simulink model "Monitor"  (R2020a)
settings: Solver=FixedStepAuto  StartTime=0.0  StopTime=4  FixedStep=0.01  RelTol=1e-3
undefined symbols (not defined in the file): a03c, a5a6, b93b39085928, BLE_Receive, Button, Case_of_study, Ci, Data_Display, Data_Display1, F4, intentBLE, Ri, Size_received, Slider, tau1
libraries: androiduilib x14, simulink x4, androidcommunicationlib x2, dspswit3 x2, hdlsllib x1
settings Model: Creator=luisi  LastModifiedBy=luisi
settings OptimizationCC: EnhancedBackFolding=on  PassReuseOutputArgsAs=Individual arguments  ZeroExternalMemoryAtStartup=off  ZeroInternalMemoryAtStartup=off  MaxStackSize=64  OptimizeBlockOrder=speed  DifferentSizesBufferReuse=on  OptimizationCustomize=off  EfficientTunableParamExpr=on
settings DebuggingCC: ParameterTunabilityLossMsg=error
settings HardwareCC: ProdBitPerPointer=32  ProdBitPerSizeT=32  ProdBitPerPtrDiffT=32  ProdLargestAtomicInteger=Long  ProdLargestAtomicFloat=Double  ProdWordSize=32  ProdHWDeviceType=ARM Compatible->ARM Cortex
settings SFSimCC: MATLABDynamicMemAlloc=off
settings RTWCC: SystemTargetFile=ert.tlc  HardwareBoard=Android Device  TemplateMakefile=ert_default_tmf  RTWVerbose=off  Toolchain=Android SDK/NDK Tools
settings CodeAppCC: ForceParamTrailComments=on  IgnoreCustomStorageClasses=off  OperatorAnnotations=on  SimulinkDataObjDesc=on  SFDataObjDesc=on  InsertBlockDesc=on
settings ERTTargetCC: SupportContinuousTime=on  ExtModeMexArgs='192.168.0.106'

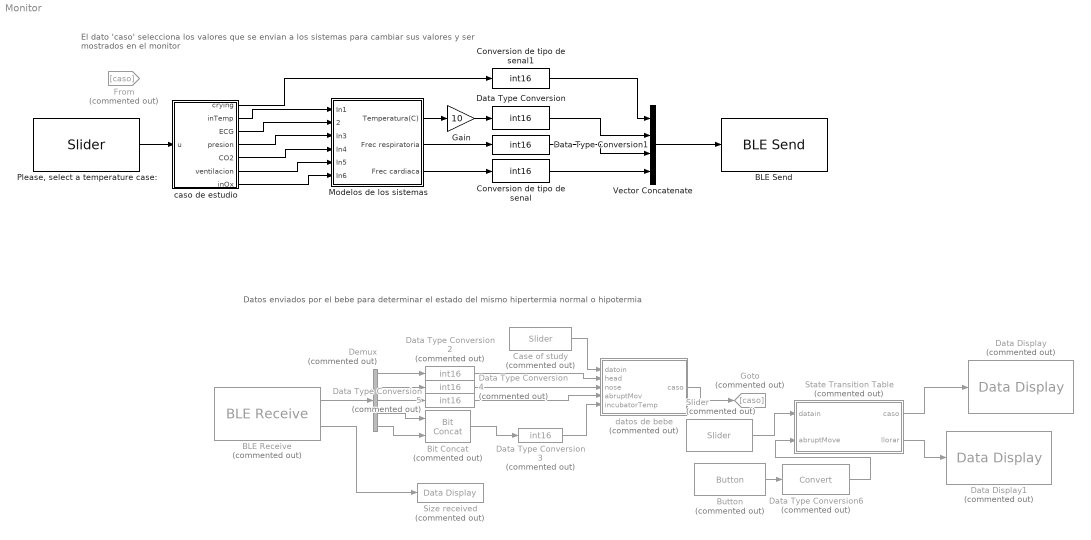
== system Monitor ==
  note: Datos enviados por el bebe para determinar el estado del mismo hipertermia normal o hipotermia
  note: El dato 'caso' selecciona los valores que se envian a los sistemas para cambiar sus valores y ser mostrados en el monitor
  BLE Receive : androidcommunicationlib/BLE Receive  Commented=on  DeviceMode=Peripheral (Server)  BluetoothAddress=62:98:F4:28:97:09  CharUUID=00002a05-0000-1000-8000-00805f9b34fb  ServiceUUID=00001801-0000-1000-8000-00805f9b34fb  device=RedmiLuisa  character=Generic Attribute\Service Changed  CustomService=on  ServiceName=Heart Rate  CharacteristicName="Heart Rate  Measurement"  CustomServiceUUID=1FFFb81d-0000-1000-8000-00805f9b34fb  CustomCharUUID=6d000000-3608-41f3-a03c-955fcbd2ea4b  DataSize=5  SampleTime=0.1  charseruuid=00001801-0000-1000-8000-00805f9b34fb\00002a05-0000-1000-8000-00805f9b34fb  seruuid=00001810-0000-1000-8000-00805f9b34fb  PeripheralService=0000180d-0000-1000-8000-00805f9b34fb  PeripheralCharacteristic=00002a37-0000-1000-8000-00805f9b34fb  chruuid=00002a37-0000-1000-8000-00805f9b34fb  BLEId=intentBLE/BLE_Receive  Devicename=RedmiLuisa  IsCustomService=0
      settings: SourceProductBaseCode=ANDROID
  BLE Send : androidcommunicationlib/BLE Send  DeviceMode=Central (Client)  BluetoothAddress=62:98:F4:28:97:09  CharUUID=6db3e235-3608-41f3-a03c-955fcbd2ea4b  ServiceUUID=1000b81d-0000-1000-8000-00805f9b34fb  device=RedmiLuisa  character=1000b81d-0000-1000-8000-00805f9b34fb\6db3e235-3608-41f3-a03c-955fcbd2ea4b  CustomService=on  ServiceName=Heart Rate  CharacteristicName="Heart Rate  Measurement"  CustomServiceUUID=0000b81d-0000-1000-8000-00805f9b34fb  CustomCharUUID=36d4dc5c-814b-4097-a5a6-b93b39085928  charseruuid=00001801-0000-1000-8000-00805f9b34fb\00002a05-0000-1000-8000-00805f9b34fb  seruuid=00001810-0000-1000-8000-00805f9b34fb  chruuid=00002a37-0000-1000-8000-00805f9b34fb  PeripheralService=0000180d-0000-1000-8000-00805f9b34fb  PeripheralCharacteristic=00002a37-0000-1000-8000-00805f9b34fb  BLEId=Monitor/BLE_Send  Devicename=RedmiLuisa  IsCustomService=0  Size=-1
      settings: SourceProductBaseCode=ANDROID
  Bit Concat : hdlsllib/Logic and Bit Operations/Bit Concat  Commented=on  numInputs=2
  Button : androiduilib/Button  Commented=on  ButtonState=Not pressed  ButtonId=intentBLE/Button  State=off  SampleTime=0.1  BlockPlatform=Android
      settings: SourceProductBaseCode=ANDROID
  Case of study : androiduilib/Slider  Commented=on  Min=0  Value=0  Max=2  Resolution=1  SliderId=intentBLE/Case_of_study  SampleTime=0.1  BlockPlatform=Android
      settings: SourceProductBaseCode=ANDROID
  Conversion de tipo de senal : DataTypeConversion  OutDataTypeStr=int16
  Conversion de tipo de senal1 : DataTypeConversion  OutDataTypeStr=int16
  Data Display : androiduilib/Data Display  Commented=on  DataDisplayId=intentBLE/Data_Display  Format=Float  Precision=6  SimulateUsing=Code generation  blockPlatform=Android
      settings: SourceProductBaseCode=ANDROID
  Data Display1 : androiduilib/Data Display  Commented=on  DataDisplayId=intentBLE/Data_Display1  Format=Float  Precision=6  SimulateUsing=Code generation  blockPlatform=Android
      settings: SourceProductBaseCode=ANDROID
  Data Type Conversion : DataTypeConversion  OutDataTypeStr=int16
  Data Type Conversion1 : DataTypeConversion  OutDataTypeStr=int16
  Data Type Conversion{2..5} (4 alike) : DataTypeConversion  Commented=on  OutDataTypeStr=int16
  Data Type Conversion6 : DataTypeConversion  Commented=on
  Demux : Demux  Commented=on  Outputs=5
  From : From  Commented=on  GotoTag=caso
  Gain : Gain  Gain=10
  Goto : Goto  Commented=on  GotoTag=caso
  Modelos de los sistemas : Subsystem
  "Please, select a temperature case:" : androiduilib/Slider  Min=0  Value=0  Max=3  Resolution=1  SliderId=Monitor/Please,_select_a_temperature_case:  SampleTime=0.1  BlockPlatform=Android
      settings: SourceProductBaseCode=ANDROID
  Size received : androiduilib/Data Display  Commented=on  DataDisplayId=intentBLE/Size_received  Format=Float  Precision=6  SimulateUsing=Code generation  blockPlatform=Android
      settings: SourceProductBaseCode=ANDROID
  Slider : androiduilib/Slider  Commented=on  Min=0  Value=0  Max=5  Resolution=1  SliderId=intentBLE/Slider  SampleTime=0.1  BlockPlatform=Android
      settings: SourceProductBaseCode=ANDROID
  State Transition Table : State Transition Table  Commented=on  TreatAsAtomicUnit=on
  Vector Concatenate : Concatenate  NumInputs=4
  caso de estudio : MATLAB Function  TreatAsAtomicUnit=on
  datos de bebe : MATLAB Function  Commented=on  TreatAsAtomicUnit=on
  wires:
  BLE Receive/2 -> Size received/1
  Case of study/1 -> datos de bebe/1(datoin)
  datos de bebe/1(caso) -> Goto/1
  caso de estudio/2(inTemp) -> Modelos de los sistemas/1(In1)
  caso de estudio/3(ECG) -> Modelos de los sistemas/2(" ")
  caso de estudio/4(presion) -> Modelos de los sistemas/3(In3)
  caso de estudio/5(CO2) -> Modelos de los sistemas/4(In4)
  caso de estudio/6(ventilacion) -> Modelos de los sistemas/5(In5)
  caso de estudio/7(inOx) -> Modelos de los sistemas/6(In6)
  Vector Concatenate/1 -> BLE Send/1
  Modelos de los sistemas/2(Frec respiratoria) -> Data Type Conversion1/1
  Modelos de los sistemas/3(Frec cardiaca) -> Conversion de tipo de senal/1
  caso de estudio/1(crying) -> Conversion de tipo de senal1/1
  Conversion de tipo de senal1/1 -> Vector Concatenate/1
  Conversion de tipo de senal/1 -> Vector Concatenate/4
  Data Type Conversion1/1 -> Vector Concatenate/3
  Data Type Conversion/1 -> Vector Concatenate/2
  Modelos de los sistemas/1(Temperatura(C)) -> Gain/1
  Gain/1 -> Data Type Conversion/1
  Bit Concat/1 -> Data Type Conversion3/1
  Demux/5 -> Bit Concat/2
  Demux/4 -> Bit Concat/1
  Demux/1 -> Data Type Conversion2/1
  BLE Receive/1 -> Demux/1
  Demux/2 -> Data Type Conversion4/1
  Data Type Conversion2/1 -> datos de bebe/2(head)
  Data Type Conversion4/1 -> datos de bebe/3(nose)
  Demux/3 -> Data Type Conversion5/1
  Data Type Conversion5/1 -> datos de bebe/4(abruptMov)
  Data Type Conversion3/1 -> datos de bebe/5(incubatorTemp)
  State Transition Table/1(caso) -> Data Display/1
  Slider/1 -> State Transition Table/1(datain)
  State Transition Table/2(llorar) -> Data Display1/1
  Button/1 -> Data Type Conversion6/1
  Data Type Conversion6/1 -> State Transition Table/2(abruptMove)
  "Please, select a temperature case:"/1 -> caso de estudio/1(u)

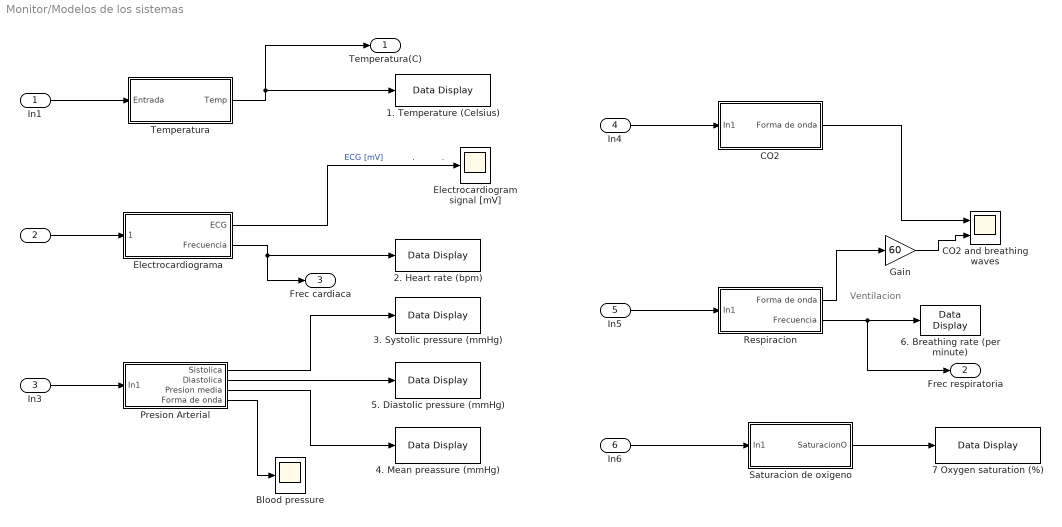
== system Monitor/Modelos de los sistemas ==
  note: Ventilacion
  In1 : Inport
  " " : Inport  Port=2
  In3 : Inport  Port=3
  In4 : Inport  Port=4
  In5 : Inport  Port=5
  In6 : Inport  Port=6
  1. Temperature (Celsius) : androiduilib/Data Display  DataDisplayId=Monitor/Modelos_de_los_sistemas/1._Temperature_(Celsius)  Format=Float  Precision=1  SimulateUsing=Code generation  blockPlatform=Android
      settings: SourceProductBaseCode=ANDROID
  2. Heart rate (bpm) : androiduilib/Data Display  DataDisplayId=Monitor/Modelos_de_los_sistemas/2._Heart_rate_(bpm)  Format=Integer  Precision=1  SimulateUsing=Code generation  blockPlatform=Android
      settings: SourceProductBaseCode=ANDROID
  3. Systolic pressure (mmHg) : androiduilib/Data Display  DataDisplayId=Monitor/Modelos_de_los_sistemas/3._Systolic_pressure_(mmHg)  Format=Integer  Precision=6  SimulateUsing=Code generation  blockPlatform=Android
      settings: SourceProductBaseCode=ANDROID
  4. Mean preassure (mmHg) : androiduilib/Data Display  DataDisplayId=Monitor/Modelos_de_los_sistemas/4._Mean_preassure_(mmHg)  Format=Integer  Precision=6  SimulateUsing=Code generation  blockPlatform=Android
      settings: SourceProductBaseCode=ANDROID
  5. Diastolic pressure (mmHg) : androiduilib/Data Display  DataDisplayId=Monitor/Modelos_de_los_sistemas/5._Diastolic_pressure_(mmHg)  Format=Integer  Precision=6  SimulateUsing=Code generation  blockPlatform=Android
      settings: SourceProductBaseCode=ANDROID
  6. Breathing rate (per minute) : androiduilib/Data Display  DataDisplayId=Monitor/Modelos_de_los_sistemas/6._Breathing_rate_(per_minute)  Format=Integer  Precision=6  SimulateUsing=Code generation  blockPlatform=Android
      settings: SourceProductBaseCode=ANDROID
  7 Oxygen saturation (%) : androiduilib/Data Display  DataDisplayId=Monitor/Modelos_de_los_sistemas/7_Oxygen_saturation_(%)  Format=Float  Precision=1  SimulateUsing=Code generation  blockPlatform=Android
      settings: SourceProductBaseCode=ANDROID
  Blood pressure : Scope
  CO2 : Subsystem
  CO2 and breathing waves : Scope  NumInputPorts=2
  Electrocardiogram signal [mV] : Scope
  Electrocardiograma : Subsystem
  Gain : Gain  Gain=60
  Presion Arterial : Subsystem
  Respiracion : Subsystem
  Saturacion de oxigeno : Subsystem
  Temperatura : Subsystem
  Temperatura(C) : Outport
  Frec respiratoria : Outport  Port=2
  Frec cardiaca : Outport  Port=3
  wires:
  In1/1 -> Temperatura/1(Entrada)
  Temperatura/1(Temp) -> Temperatura(C)/1, 1. Temperature (Celsius)/1
  Presion Arterial/2(Diastolica) -> 5. Diastolic pressure (mmHg)/1
  Presion Arterial/3(Presion media) -> 4. Mean preassure (mmHg)/1
  Presion Arterial/1(Sistolica) -> 3. Systolic pressure (mmHg)/1
  In5/1 -> Respiracion/1(In1)
  In3/1 -> Presion Arterial/1(In1)
  In4/1 -> CO2/1(In1)
  Respiracion/2(Frecuencia) -> Frec respiratoria/1, 6. Breathing rate (per minute)/1
  Electrocardiograma/2(Frecuencia) -> Frec cardiaca/1, 2. Heart rate (bpm)/1
  CO2/1(Forma de onda) -> CO2 and breathing waves/1
  Respiracion/1(Forma de onda) -> Gain/1
  Gain/1 -> CO2 and breathing waves/2
  Presion Arterial/4(Forma de onda) -> Blood pressure/1
  Electrocardiograma/1(ECG) -> Electrocardiogram signal [mV]/1  "ECG [mV]           .          ."
  Saturacion de oxigeno/1(SaturacionO) -> 7 Oxygen saturation (%)/1
  In6/1 -> Saturacion de oxigeno/1(In1)
  " "/1 -> Electrocardiograma/1(" ")

== system Monitor/Modelos de los sistemas/CO2 ==
  In1 : Inport
  Constant3 : Constant  Value=0
  Demux : Demux  Outputs=2
  Subsystem1 : Subsystem
  Switch : Switch  Criteria=u2 > Threshold
  Transfer Fcn1 : TransferFcn  Denominator=[tau1 1]
  Forma de onda : Outport
  wires:
  In1/1 -> Demux/1
  Demux/1 -> [phi]
  Demux/2 -> [tf]
  Constant3/1 -> Switch/1
  Subsystem1/1(Out1) -> Switch/2
  Switch/1 -> Transfer Fcn1/1
  [tf] -> Subsystem1/1(In1)
  [phi] -> Switch/3
  Transfer Fcn1/1 -> Forma de onda/1

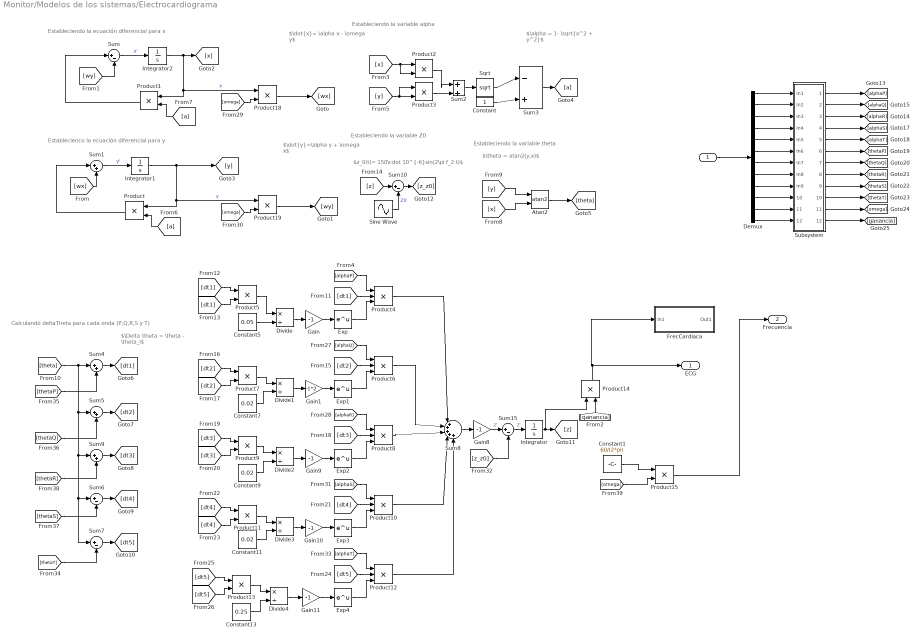
== system Monitor/Modelos de los sistemas/Electrocardiograma ==
  note: $\dot{y}=\alpha y + \omega x$
  note: $\dot{x}= \alpha x - \omega y$
  note: $\alpha = 1- \sqrt{x^2 + y^2}$
  note: $z_0(t)= 150\cdot 10^{-6}sin(2\pi f_2 t)$
  note: Estableciendo la ecuación diferencial para x
  note: Estableciendo la variable alpha
  note: Establecienco la ecuación diferencial para y
  note: Estableciendo la variable theta
  note: Estableciendo la variable Z0
  note: $\theta = atan2(y,x)$
  note: Calculando deltaTheta para cada onda (P,Q,R,S y T)
  note: $\Delta \theta = \theta - \theta_i$
  " " : Inport
  Atan2 : Trigonometry  Operator=atan2
  Constant : Constant
  Constant1 : Constant  Value=60/(2*pi)
  Constant11 : Constant  Value=0.02
  Constant13 : Constant  Value=0.25
  Constant5 : Constant  Value=0.05
  Constant7 : Constant  Value=0.02
  Constant9 : Constant  Value=0.02
  Demux : Demux  Outputs=12
  Divide{,1..4} (5 alike) : Product  Inputs=*/
  Exp{,1..4} (5 alike) : Math  SaturateOnIntegerOverflow=on
  FrecCardiaca : Subsystem
  Gain{,8..11} (5 alike) : Gain  Gain=-1
  Gain1 : Gain  Gain=-1*2
  Integrator : Integrator  InitialCondition=1000
  Integrator1 : Integrator
  Integrator2 : Integrator  InitialCondition=2
  Product{,1..3,5,7,9,11,13..15,18..19} (13 alike) : Product
  Product{4,6,8,10,12} (5 alike) : Product  Inputs=3
  Sine Wave : Sin  Amplitude=0.15e-3  Frequency=0.25  SampleTime=0
  Sqrt : Sqrt  SaturateOnIntegerOverflow=on
  Subsystem : Subsystem
  Sum{,6..7,10,15} (5 alike) : Sum  Inputs=|+-
  Sum{1..2,4..5,9} (5 alike) : Sum  Inputs=|++
  Sum3 : Sum  Inputs=|-+
  Sum8 : Sum  Inputs=|+++++
  ECG : Outport
  Frecuencia : Outport  Port=2
  wires:
  [dt2] -> Product6/2
  Product4/1 -> Sum8/1
  [x] -> Atan2/2
  Product3/1 -> Sum2/2
  [y] -> Atan2/1
  Product/1 -> Sum1/1
  Product5/1 -> Divide/1
  [dt2] -> Product7/2
  Gain/1 -> Exp/1
  Product1/1 -> Sum/1
  Constant/1 -> Sum3/2
  Divide1/1 -> Gain1/1
  Exp4/1 -> Product12/3
  Exp3/1 -> Product10/3
  Gain11/1 -> Exp4/1
  Exp/1 -> Product4/3
  [alphaT] -> Product12/1
  Constant11/1 -> Divide3/2
  Divide2/1 -> Gain9/1
  [dt1] -> Product4/2
  Product18/1 -> [wx]
  Sum2/1 -> Sqrt/1
  [a] -> Product1/2
  [thetaP] -> Sum4/2
  Product8/1 -> Sum8/3
  Exp2/1 -> Product8/3
  Product11/1 -> Divide3/1
  [dt3] -> Product9/2
  Integrator1/1 -> [y], Product19/1, Product/1  "y"
  Constant5/1 -> Divide/2
  Product7/1 -> Divide1/1
  [dt4] -> Product11/1
  Sqrt/1 -> Sum3/1
  Product13/1 -> Divide4/1
  Gain10/1 -> Exp3/1
  [dt1] -> Product5/1
  Gain1/1 -> Exp1/1
  [dt5] -> Product13/2
  [dt4] -> Product11/2
  [dt1] -> Product5/2
  Constant9/1 -> Divide2/2
  [dt5] -> Product12/2
  Divide/1 -> Gain/1
  Divide4/1 -> Gain11/1
  [dt5] -> Product13/1
  Product12/1 -> Sum8/5
  Product6/1 -> Sum8/2
  Constant13/1 -> Divide4/2
  Product10/1 -> Sum8/4
  Sum5/1 -> [dt2]
  [dt4] -> Product10/2
  Sine Wave/1 -> Sum10/2  "Z0"
  Sum6/1 -> [dt4]
  Sum1/1 -> Integrator1/1  "y'"
  [dt3] -> Product9/1
  Atan2/1 -> [theta]
  [omega] -> Product19/2
  Sum7/1 -> [dt5]
  Sum10/1 -> [z_z0]
  Gain8/1 -> Sum15/1  "z'"
  Integrator/1 -> Product14/1, [z]
  [dt3] -> Product8/2
  [theta] -> Sum7/1, Sum6/1, Sum9/1, Sum5/1, Sum4/1
  [z_z0] -> Sum15/2
  [a] -> Product/2
  Integrator2/1 -> [x], Product1/1, Product18/1  "x"
  Exp1/1 -> Product6/3
  [thetaS] -> Sum6/2
  Sum4/1 -> [dt1]
  [alphaP] -> Product4/1
  Sum15/1 -> Integrator/1  "z'"
  Product19/1 -> [wy]
  Sum/1 -> Integrator2/1  "x'"
  [wx] -> Sum1/2
  [thetaT] -> Sum7/2
  [y] -> Product3/1, Product3/2
  [wy] -> Sum/2
  [thetaQ] -> Sum5/2
  Product9/1 -> Divide2/1
  Constant7/1 -> Divide1/2
  Sum3/1 -> [a]
  [x] -> Product2/2, Product2/1
  [dt2] -> Product7/1
  [z] -> Sum10/1
  Gain9/1 -> Exp2/1
  [omega] -> Product18/2
  Product2/1 -> Sum2/1
  Product14/1 -> FrecCardiaca/1(In1), ECG/1
  Divide3/1 -> Gain10/1
  Sum8/1 -> Gain8/1
  " "/1 -> Demux/1
  [ganancia] -> Product14/2
  [alphaS] -> Product10/1
  [alphaR] -> Product8/1
  [alphaQ] -> Product6/1
  Sum9/1 -> [dt3]
  [thetaR] -> Sum9/2
  [omega] -> Product15/2
  Constant1/1 -> Product15/1
  Product15/1 -> Frecuencia/1
  Demux/1 -> Subsystem/1(In1)
  Demux/2 -> Subsystem/2(In2)
  Demux/3 -> Subsystem/3(In3)
  Demux/4 -> Subsystem/4(In4)
  Demux/5 -> Subsystem/5(In5)
  Demux/6 -> Subsystem/6(In6)
  Demux/7 -> Subsystem/7(In7)
  Demux/8 -> Subsystem/8(In8)
  Demux/9 -> Subsystem/9(In9)
  Demux/10 -> Subsystem/10(In10)
  Demux/11 -> Subsystem/11(In11)
  Demux/12 -> Subsystem/12(In12)
  Subsystem/6(Out6) -> [thetaP]
  Subsystem/5(Out5) -> [alphaT]
  Subsystem/7(Out7) -> [thetaQ]
  Subsystem/8(Out8) -> [thetaR]
  Subsystem/9(Out9) -> [thetaS]
  Subsystem/10(Out10) -> [thetaT]
  Subsystem/11(Out11) -> [omega]
  Subsystem/12(Out12) -> [ganancia]
  Subsystem/1(Out1) -> [alphaP]
  Subsystem/2(Out2) -> [alphaQ]
  Subsystem/3(Out3) -> [alphaR]
  Subsystem/4(Out4) -> [alphaS]

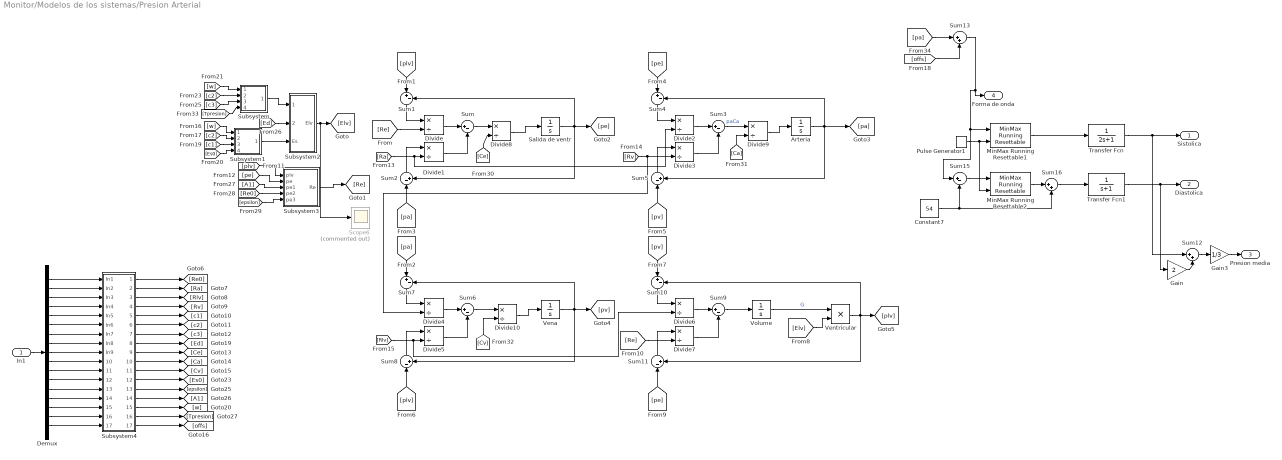
== system Monitor/Modelos de los sistemas/Presion Arterial ==
  In1 : Inport
  Arteria : Integrator  InitialCondition=70
  Constant7 : Constant  Value=54
  Demux : Demux  Outputs=17
  Divide{,1..10} (11 alike) : Product  Inputs=*/
  Gain : Gain  Gain=2
  Gain3 : Gain  Gain=1/3
  MinMax Running Resettable1 : simulink/Math Operations/MinMax Running Resettable  Function=max  vinit=40
  MinMax Running Resettable2 : simulink/Math Operations/MinMax Running Resettable  Function=min  vinit=0.0
  Pulse Generator1 : DiscretePulseGenerator  PulseType=Time based  Period=8  PulseWidth=0.5
  Salida de ventr : Integrator  InitialCondition=49.896
  Scope6 : Scope  Commented=on
  Subsystem : Subsystem
  Subsystem1 : Subsystem
  Subsystem2 : Subsystem
  Subsystem3 : Subsystem
  Subsystem4 : Subsystem
  Sum{,1,3..4,6..7,9..10,15} (9 alike) : Sum  Inputs=|+-
  Sum{2,5,8,11} (4 alike) : Sum  Inputs=|-+
  Sum12 : Sum  Inputs=|++
  Sum13 : Sum  Inputs=|++
  Sum16 : Sum  Inputs=|++
  Transfer Fcn : TransferFcn  Denominator=[2 1]
  Transfer Fcn1 : TransferFcn  Denominator=[1 1]
  Vena : Integrator  InitialCondition=16.628
  Ventricular : Product
  Volume : Integrator  InitialCondition=49.714/0.0655
  Sistolica : Outport
  Diastolica : Outport  Port=2
  Presion media : Outport  Port=3
  Forma de onda : Outport  Port=4
  wires:
  Gain3/1 -> Presion media/1
  Sum16/1 -> Transfer Fcn1/1
  MinMax Running Resettable2/1 -> Sum16/1
  Sum3/1 -> Divide9/1  "paCa"
  Sum10/1 -> Divide6/1
  MinMax Running Resettable1/1 -> Transfer Fcn/1
  Subsystem2/1(Elv) -> Scope6/1, [Elv]
  Constant7/1 -> Sum16/2, Sum15/2
  Salida de ventr/1 -> [pe], Sum2/2, Sum1/2
  Sum13/1 -> Forma de onda/1, Sum15/1, MinMax Running Resettable1/1
  Divide6/1 -> Sum9/1
  Pulse Generator1/1 -> MinMax Running Resettable2/2, MinMax Running Resettable1/2
  [Elv] -> Ventricular/2
  Divide8/1 -> Salida de ventr/1
  [Re] -> Divide/2
  [Rv] -> Divide4/2, Divide3/2
  Sum5/1 -> Divide3/1
  [plv] -> Subsystem3/1(plv)
  Divide/1 -> Sum/1
  [plv] -> Sum1/1
  [pv] -> Sum10/1
  Ventricular/1 -> Sum10/2, [plv], Sum11/2
  Sum15/1 -> MinMax Running Resettable2/1
  [pe] -> Sum4/1
  [pe] -> Subsystem3/2(pe)
  Sum9/1 -> Volume/1
  [plv] -> Sum8/1
  Divide10/1 -> Vena/1
  [pv] -> Sum5/1
  Divide7/1 -> Sum9/2
  [Rlv] -> Divide6/2, Divide5/2
  Divide9/1 -> Arteria/1
  Sum8/1 -> Divide5/1
  Sum11/1 -> Divide7/1
  Divide2/1 -> Sum3/1
  [pe] -> Sum11/1
  [pa] -> Sum7/1
  Sum7/1 -> Divide4/1
  Vena/1 -> [pv], Sum8/2, Sum7/2
  Divide3/1 -> Sum3/2
  Sum6/1 -> Divide10/1
  Volume/1 -> Ventricular/1  "G"
  Divide5/1 -> Sum6/2
  Divide4/1 -> Sum6/1
  Arteria/1 -> Sum5/2, Sum4/2, [pa]
  [pa] -> Sum2/1
  [Re] -> Divide7/2
  Sum2/1 -> Divide1/1
  Sum1/1 -> Divide/1
  Sum/1 -> Divide8/1
  Sum4/1 -> Divide2/1
  Subsystem3/1(Re) -> [Re]
  Subsystem/1(alphat) -> Subsystem2/1(alpha)
  Subsystem1/1(E_s) -> Subsystem2/3(Es)
  Divide1/1 -> Sum/2
  [Ra] -> Divide2/2, Divide1/2
  In1/1 -> Demux/1
  [w] -> Subsystem1/1(In1)
  [c2] -> Subsystem1/2(In2)
  [c1] -> Subsystem1/3(In3)
  [Es0] -> Subsystem1/4(In4)
  [w] -> Subsystem/1(In1)
  [c2] -> Subsystem/2(In2)
  [c3] -> Subsystem/3(In3)
  [Ed] -> Subsystem2/2(In2)
  [A1] -> Subsystem3/3(pe1)
  [Re0] -> Subsystem3/4(pe2)
  [epsilon] -> Subsystem3/5(pe3)
  [Ce] -> Divide8/2
  [Ca] -> Divide9/2
  [Cv] -> Divide10/2
  [Tpresion] -> Subsystem/4(In4)
  Sum12/1 -> Gain3/1
  Gain/1 -> Sum12/2
  Transfer Fcn/1 -> Sum12/1, Sistolica/1
  Transfer Fcn1/1 -> Gain/1, Diastolica/1
  [offs] -> Sum13/2
  [pa] -> Sum13/1
  Demux/1 -> Subsystem4/1(In1)
  Demux/2 -> Subsystem4/2(In2)
  Demux/3 -> Subsystem4/3(In3)
  Demux/4 -> Subsystem4/4(In4)
  Demux/5 -> Subsystem4/5(In5)
  Demux/6 -> Subsystem4/6(In6)
  Demux/7 -> Subsystem4/7(In7)
  Demux/8 -> Subsystem4/8(In8)
  Demux/9 -> Subsystem4/9(In9)
  Demux/10 -> Subsystem4/10(In10)
  Demux/11 -> Subsystem4/11(In11)
  Demux/12 -> Subsystem4/12(In12)
  Demux/13 -> Subsystem4/13(In13)
  Demux/14 -> Subsystem4/14(In14)
  Demux/15 -> Subsystem4/15(In15)
  Demux/16 -> Subsystem4/16(In16)
  Demux/17 -> Subsystem4/17(In17)
  Subsystem4/7(Out7) -> [c3]
  Subsystem4/1(Out1) -> [Re0]
  Subsystem4/2(Out2) -> [Ra]
  Subsystem4/3(Out3) -> [Rlv]
  Subsystem4/4(Out4) -> [Rv]
  Subsystem4/5(Out5) -> [c1]
  Subsystem4/6(Out6) -> [c2]
  Subsystem4/8(Out8) -> [Ed]
  Subsystem4/9(Out9) -> [Ce]
  Subsystem4/10(Out10) -> [Ca]
  Subsystem4/11(Out11) -> [Cv]
  Subsystem4/12(Out12) -> [Es0]
  Subsystem4/13(Out13) -> [epsilon]
  Subsystem4/14(Out14) -> [A1]
  Subsystem4/15(Out15) -> [w]
  Subsystem4/16(Out16) -> [Tpresion]
  Subsystem4/17(Out17) -> [offs]

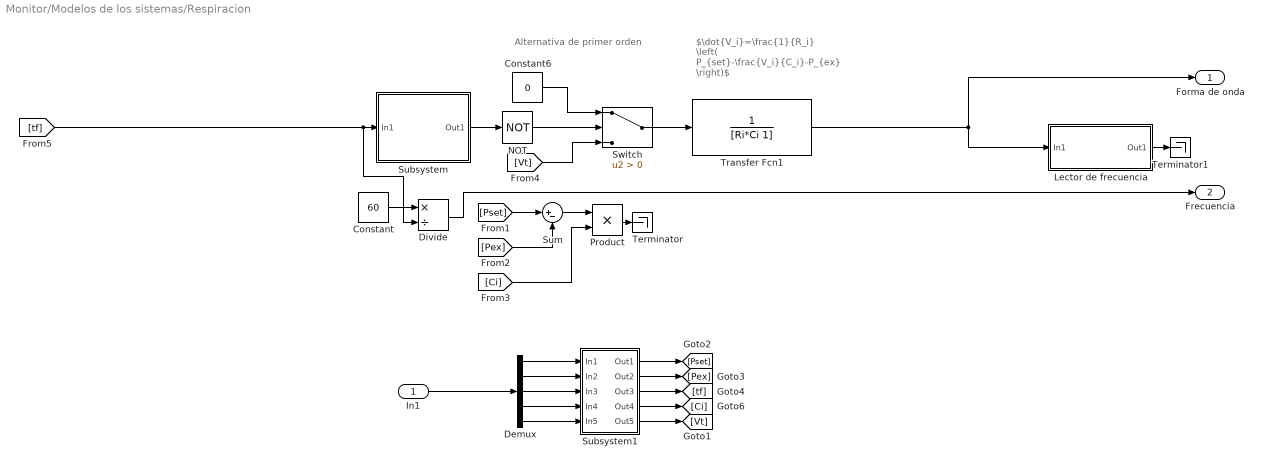
== system Monitor/Modelos de los sistemas/Respiracion ==
  note: $\dot{V_i}=\frac{1}{R_i} \left( P_{set}-\frac{V_i}{C_i}-P_{ex} \right)$
  note: Alternativa de primer orden
  In1 : Inport
  Constant : Constant  Value=60
  Constant6 : Constant  Value=0
  Demux : Demux  Outputs=5
  Divide : Product  Inputs=*/
  Lector de frecuencia : Subsystem
  NOT : Logic  Operator=NOT  IconShape=distinctive  AllPortsSameDT=off  OutDataTypeStr=boolean
  Product : Product
  Subsystem : Subsystem
  Subsystem1 : Subsystem
  Sum : Sum  Inputs=|+-
  Switch : Switch  Criteria=u2 > Threshold
  Terminator : Terminator
  Terminator1 : Terminator
  Transfer Fcn1 : TransferFcn  Denominator=[Ri*Ci 1]
  Forma de onda : Outport
  Frecuencia : Outport  Port=2
  wires:
  In1/1 -> Demux/1
  Transfer Fcn1/1 -> Forma de onda/1, Lector de frecuencia/1(In1)
  [Ci] -> Product/2
  Switch/1 -> Transfer Fcn1/1
  Sum/1 -> Product/1
  Product/1 -> Terminator/1
  [Vt] -> Switch/3
  [Pex] -> Sum/2
  Constant6/1 -> Switch/1
  [Pset] -> Sum/1
  NOT/1 -> Switch/2
  Subsystem/1(Out1) -> NOT/1
  Constant/1 -> Divide/1
  Divide/1 -> Frecuencia/1
  Lector de frecuencia/1(Out1) -> Terminator1/1
  [tf] -> Divide/2, Subsystem/1(In1)
  Demux/1 -> Subsystem1/1(In1)
  Demux/2 -> Subsystem1/2(In2)
  Demux/3 -> Subsystem1/3(In3)
  Demux/4 -> Subsystem1/4(In4)
  Demux/5 -> Subsystem1/5(In5)
  Subsystem1/1(Out1) -> [Pset]
  Subsystem1/2(Out2) -> [Pex]
  Subsystem1/3(Out3) -> [tf]
  Subsystem1/4(Out4) -> [Ci]
  Subsystem1/5(Out5) -> [Vt]

== system Monitor/Modelos de los sistemas/Saturacion de oxigeno ==
  In1 : Inport
  Data Type Conversion : DataTypeConversion
  Subsystem4 : Subsystem
  Transfer Fcn : TransferFcn  Numerator=95.4  Denominator=[0.4 1]
  SaturacionO : Outport
  wires:
  Data Type Conversion/1 -> Transfer Fcn/1
  Transfer Fcn/1 -> SaturacionO/1
  Subsystem4/1(Out1) -> Data Type Conversion/1
  In1/1 -> Subsystem4/1(In1)

== system Monitor/Modelos de los sistemas/Temperatura ==
  Entrada : Inport
  Data Type Conversion : DataTypeConversion
  Sine Wave : Sin  Amplitude=0.005  Frequency=0.1  SampleTime=0
  Sum : Sum  Inputs=|++
  Transfer Fcn : TransferFcn  Numerator=36.3  Denominator=[1 1]
  Temp : Outport
  wires:
  Data Type Conversion/1 -> Transfer Fcn/1
  Transfer Fcn/1 -> Temp/1
  Entrada/1 -> Sum/1
  Sine Wave/1 -> Sum/2
  Sum/1 -> Data Type Conversion/1

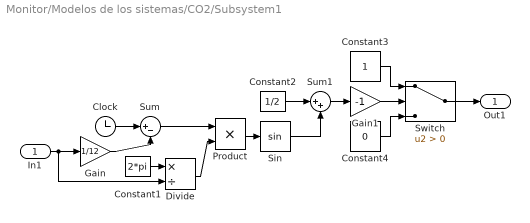
== system Monitor/Modelos de los sistemas/CO2/Subsystem1 ==
  In1 : Inport
  Clock : Clock
  Constant1 : Constant  Value=2*pi
  Constant2 : Constant  Value=1/2
  Constant3 : Constant
  Constant4 : Constant  Value=0
  Divide : Product  Inputs=*/
  Gain : Gain  Gain=1/12
  Gain1 : Gain  Gain=-1
  Product : Product
  Sin : Trigonometry
  Sum : Sum  Inputs=|+-
  Sum1 : Sum  Inputs=|++
  Switch : Switch  Criteria=u2 > Threshold
  Out1 : Outport
  wires:
  Constant1/1 -> Divide/1
  Divide/1 -> Product/2
  Constant2/1 -> Sum1/1
  Sum/1 -> Product/1
  Gain/1 -> Sum/2
  Constant3/1 -> Switch/1
  Sum1/1 -> Gain1/1
  Sin/1 -> Sum1/2
  Constant4/1 -> Switch/3
  Gain1/1 -> Switch/2
  Product/1 -> Sin/1
  In1/1 -> Divide/2, Gain/1
  Clock/1 -> Sum/1
  Switch/1 -> Out1/1

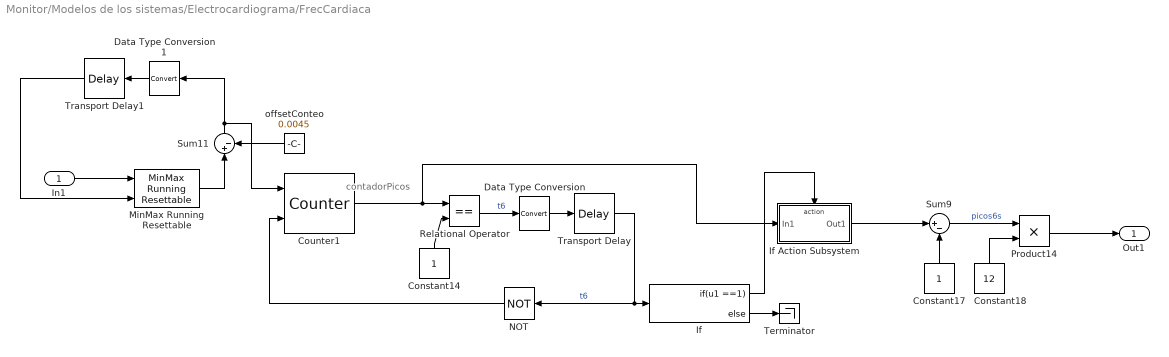
== system Monitor/Modelos de los sistemas/Electrocardiograma/FrecCardiaca ==
  note: contadorPicos
  In1 : Inport
  Constant14 : Constant
  Constant17 : Constant
  Constant18 : Constant  Value=12
  Counter1 : dspswit3/Counter  Direction=Up  CountEvent=Rising edge  CounterSize=User defined  MaxCount=100  InitialCount=0  Output=Count  HitValue=32  ResetInput=on  SamplesPerFrame=1  Ts=1  CntDtype=double  HitDtype=Logical
  Data Type Conversion : DataTypeConversion
  Data Type Conversion1 : DataTypeConversion
  If : If  IfExpression=u1 ==1
  If Action Subsystem : Subsystem  TreatAsAtomicUnit=on
  MinMax Running Resettable : simulink/Math Operations/MinMax Running Resettable  Function=max  vinit=0.0045
  NOT : Logic  Operator=NOT  IconShape=distinctive  AllPortsSameDT=off  OutDataTypeStr=boolean
  Product14 : Product
  Relational Operator : RelationalOperator  Operator===  OutDataTypeStr=boolean  RndMeth=Simplest
  Sum11 : Sum  Inputs=|+-
  Sum9 : Sum  Inputs=|+-
  Terminator : Terminator
  Transport Delay : TransportDelay  DelayTime=5
  Transport Delay1 : TransportDelay  DelayTime=0.16
  offsetConteo : Constant  Value=0.0045
  Out1 : Outport
  wires:
  NOT/1 -> Counter1/2
  Sum9/1 -> Product14/1  "picos6s"
  If/2 -> Terminator/1
  Product14/1 -> Out1/1
  If Action Subsystem/1(Out1) -> Sum9/1
  If/1 -> If Action Subsystem/Action
  Transport Delay/1 -> NOT/1, If/1  "t6"
  Constant17/1 -> Sum9/2
  Constant14/1 -> Relational Operator/2
  In1/1 -> MinMax Running Resettable/1
  Counter1/1 -> If Action Subsystem/1(In1), Relational Operator/1
  MinMax Running Resettable/1 -> Sum11/1
  offsetConteo/1 -> Sum11/2
  Constant18/1 -> Product14/2
  Transport Delay1/1 -> MinMax Running Resettable/2
  Sum11/1 -> Data Type Conversion1/1, Counter1/1
  Relational Operator/1 -> Data Type Conversion/1  "t6"
  Data Type Conversion/1 -> Transport Delay/1
  Data Type Conversion1/1 -> Transport Delay1/1

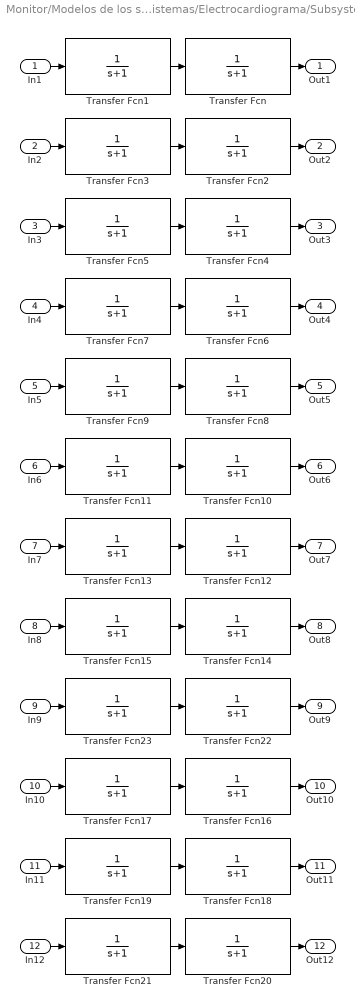
== system Monitor/Modelos de los sistemas/Electrocardiograma/Subsystem ==
  In1 : Inport
  In2 : Inport  Port=2
  In3 : Inport  Port=3
  In4 : Inport  Port=4
  In5 : Inport  Port=5
  In6 : Inport  Port=6
  In7 : Inport  Port=7
  In8 : Inport  Port=8
  In9 : Inport  Port=9
  In10 : Inport  Port=10
  In11 : Inport  Port=11
  In12 : Inport  Port=12
  Transfer Fcn{,1..23} (24 alike) : TransferFcn  Numerator=1  Denominator=[1 1]
  Out1 : Outport
  Out2 : Outport  Port=2
  Out3 : Outport  Port=3
  Out4 : Outport  Port=4
  Out5 : Outport  Port=5
  Out6 : Outport  Port=6
  Out7 : Outport  Port=7
  Out8 : Outport  Port=8
  Out9 : Outport  Port=9
  Out10 : Outport  Port=10
  Out11 : Outport  Port=11
  Out12 : Outport  Port=12
  wires:
  Transfer Fcn1/1 -> Transfer Fcn/1
  In1/1 -> Transfer Fcn1/1
  Transfer Fcn/1 -> Out1/1
  Transfer Fcn2/1 -> Out2/1
  In2/1 -> Transfer Fcn3/1
  Transfer Fcn3/1 -> Transfer Fcn2/1
  Transfer Fcn7/1 -> Transfer Fcn6/1
  In4/1 -> Transfer Fcn7/1
  Transfer Fcn6/1 -> Out4/1
  Transfer Fcn4/1 -> Out3/1
  In3/1 -> Transfer Fcn5/1
  Transfer Fcn5/1 -> Transfer Fcn4/1
  Transfer Fcn8/1 -> Out5/1
  In8/1 -> Transfer Fcn15/1
  Transfer Fcn15/1 -> Transfer Fcn14/1
  In7/1 -> Transfer Fcn13/1
  Transfer Fcn12/1 -> Out7/1
  Transfer Fcn14/1 -> Out8/1
  Transfer Fcn11/1 -> Transfer Fcn10/1
  Transfer Fcn10/1 -> Out6/1
  Transfer Fcn9/1 -> Transfer Fcn8/1
  In6/1 -> Transfer Fcn11/1
  In5/1 -> Transfer Fcn9/1
  Transfer Fcn13/1 -> Transfer Fcn12/1
  Transfer Fcn19/1 -> Transfer Fcn18/1
  In9/1 -> Transfer Fcn23/1
  In10/1 -> Transfer Fcn17/1
  Transfer Fcn23/1 -> Transfer Fcn22/1
  Transfer Fcn16/1 -> Out10/1
  Transfer Fcn17/1 -> Transfer Fcn16/1
  Transfer Fcn20/1 -> Out12/1
  Transfer Fcn18/1 -> Out11/1
  In11/1 -> Transfer Fcn19/1
  Transfer Fcn21/1 -> Transfer Fcn20/1
  In12/1 -> Transfer Fcn21/1
  Transfer Fcn22/1 -> Out9/1

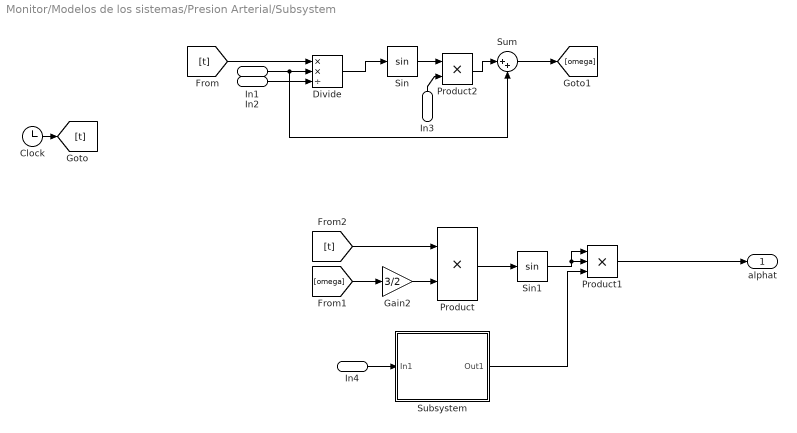
== system Monitor/Modelos de los sistemas/Presion Arterial/Subsystem ==
  In1 : Inport
  In2 : Inport  Port=2
  In3 : Inport  Port=3
  In4 : Inport  Port=4
  Clock : Clock
  Divide : Product  Inputs=**/
  Gain2 : Gain  Gain=3/2
  Product : Product
  Product1 : Product  Inputs=3
  Product2 : Product
  Sin : Trigonometry
  Sin1 : Trigonometry
  Subsystem : Subsystem
  Sum : Sum  Inputs=|++
  alphat : Outport
  wires:
  Clock/1 -> [t]
  [t] -> Divide/1
  Divide/1 -> Sin/1
  Sin/1 -> Product2/1
  Product2/1 -> Sum/1
  In1/1 -> Sum/2, Divide/2
  Sum/1 -> [omega]
  [t] -> Product/1
  [omega] -> Gain2/1
  Product/1 -> Sin1/1
  Sin1/1 -> Product1/1, Product1/2
  Product1/1 -> alphat/1
  Gain2/1 -> Product/2
  Subsystem/1(Out1) -> Product1/3
  In2/1 -> Divide/3
  In3/1 -> Product2/2
  In4/1 -> Subsystem/1(In1)

== system Monitor/Modelos de los sistemas/Presion Arterial/Subsystem1 ==
  In1 : Inport
  In2 : Inport  Port=2
  In3 : Inport  Port=3
  In4 : Inport  Port=4
  Clock : Clock
  Divide : Product  Inputs=**/
  Product : Product
  Sin : Trigonometry
  Sum : Sum  Inputs=|++
  E_s : Outport
  wires:
  Sum/1 -> E_s/1
  In4/1 -> Sum/2
  Product/1 -> Sum/1
  Sin/1 -> Product/1
  Divide/1 -> Sin/1
  [t] -> Divide/1
  Clock/1 -> [t]
  In2/1 -> Divide/3
  In1/1 -> Divide/2
  In3/1 -> Product/2

== system Monitor/Modelos de los sistemas/Presion Arterial/Subsystem2 ==
  alpha : Inport
  In2 : Inport  Port=2
  Es : Inport  Port=3
  Product : Product
  Sum : Sum
  Sum1 : Sum  Inputs=-+
  Elv : Outport
  wires:
  In2/1 -> Sum1/1, Sum/1
  Es/1 -> Sum1/2
  alpha/1 -> Product/2
  Sum1/1 -> Product/1
  Product/1 -> Sum/2
  Sum/1 -> Elv/1

== system Monitor/Modelos de los sistemas/Presion Arterial/Subsystem3 ==
  plv : Inport
  pe : Inport  Port=2
  pe1 : Inport  Port=3
  pe2 : Inport  Port=4
  pe3 : Inport  Port=5
  Constant : Constant
  Exp : Math  SaturateOnIntegerOverflow=on
  Gain3 : Gain  Gain=-1
  Product : Product
  Product1 : Product
  Product2 : Product
  Sum : Sum
  Sum1 : Sum  Inputs=+-
  Re : Outport
  wires:
  Sum/1 -> Product1/1
  Product1/1 -> Re/1
  Constant/1 -> Sum/1
  Product2/1 -> Sum/2
  Exp/1 -> Product2/1
  plv/1 -> Sum1/1
  pe/1 -> Sum1/2
  Product/1 -> Exp/1
  Sum1/1 -> Product/1
  pe1/1 -> Gain3/1
  Gain3/1 -> Product/2
  pe2/1 -> Product1/2
  pe3/1 -> Product2/2

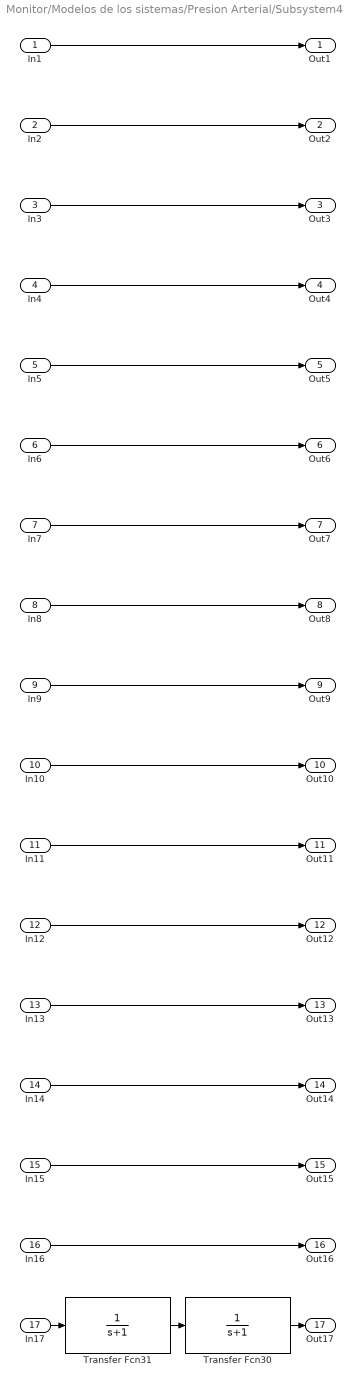
== system Monitor/Modelos de los sistemas/Presion Arterial/Subsystem4 ==
  In1 : Inport
  In2 : Inport  Port=2
  In3 : Inport  Port=3
  In4 : Inport  Port=4
  In5 : Inport  Port=5
  In6 : Inport  Port=6
  In7 : Inport  Port=7
  In8 : Inport  Port=8
  In9 : Inport  Port=9
  In10 : Inport  Port=10
  In11 : Inport  Port=11
  In12 : Inport  Port=12
  In13 : Inport  Port=13
  In14 : Inport  Port=14
  In15 : Inport  Port=15
  In16 : Inport  Port=16
  In17 : Inport  Port=17
  Transfer Fcn30 : TransferFcn  Numerator=1  Denominator=[1 1]
  Transfer Fcn31 : TransferFcn  Numerator=1  Denominator=[1 1]
  Out1 : Outport
  Out2 : Outport  Port=2
  Out3 : Outport  Port=3
  Out4 : Outport  Port=4
  Out5 : Outport  Port=5
  Out6 : Outport  Port=6
  Out7 : Outport  Port=7
  Out8 : Outport  Port=8
  Out9 : Outport  Port=9
  Out10 : Outport  Port=10
  Out11 : Outport  Port=11
  Out12 : Outport  Port=12
  Out13 : Outport  Port=13
  Out14 : Outport  Port=14
  Out15 : Outport  Port=15
  Out16 : Outport  Port=16
  Out17 : Outport  Port=17
  wires:
  In1/1 -> Out1/1
  In2/1 -> Out2/1
  In4/1 -> Out4/1
  In3/1 -> Out3/1
  In5/1 -> Out5/1
  In7/1 -> Out7/1
  In8/1 -> Out8/1
  In6/1 -> Out6/1
  In10/1 -> Out10/1
  In12/1 -> Out12/1
  In11/1 -> Out11/1
  In9/1 -> Out9/1
  Transfer Fcn31/1 -> Transfer Fcn30/1
  In14/1 -> Out14/1
  In16/1 -> Out16/1
  Transfer Fcn30/1 -> Out17/1
  In13/1 -> Out13/1
  In17/1 -> Transfer Fcn31/1
  In15/1 -> Out15/1

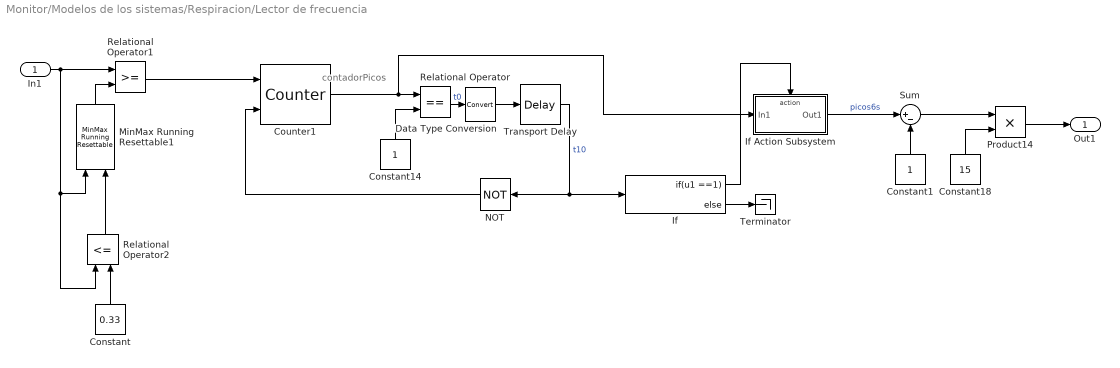
== system Monitor/Modelos de los sistemas/Respiracion/Lector de frecuencia ==
  note: contadorPicos
  In1 : Inport
  Constant : Constant  Value=0.33
  Constant1 : Constant
  Constant14 : Constant
  Constant18 : Constant  Value=15
  Counter1 : dspswit3/Counter  Direction=Up  CountEvent=Rising edge  CounterSize=User defined  MaxCount=100  InitialCount=0  Output=Count  HitValue=32  ResetInput=on  SamplesPerFrame=1  Ts=1  CntDtype=double  HitDtype=Logical
  Data Type Conversion : DataTypeConversion
  If : If  IfExpression=u1 ==1
  If Action Subsystem : Subsystem  TreatAsAtomicUnit=on
  MinMax Running Resettable1 : simulink/Math Operations/MinMax Running Resettable  Function=max  vinit=0.33
  NOT : Logic  Operator=NOT  IconShape=distinctive  AllPortsSameDT=off  OutDataTypeStr=boolean
  Product14 : Product
  Relational Operator : RelationalOperator  Operator===  OutDataTypeStr=boolean  RndMeth=Simplest
  Relational Operator1 : RelationalOperator  OutDataTypeStr=boolean  RndMeth=Simplest
  Relational Operator2 : RelationalOperator  Operator=<=  OutDataTypeStr=boolean  RndMeth=Simplest
  Sum : Sum  Inputs=|+-
  Terminator : Terminator
  Transport Delay : TransportDelay  DelayTime=4
  Out1 : Outport
  wires:
  Relational Operator1/1 -> Counter1/1
  Product14/1 -> Out1/1
  If/2 -> Terminator/1
  Constant18/1 -> Product14/2
  Transport Delay/1 -> NOT/1, If/1  "t10"
  NOT/1 -> Counter1/2
  Counter1/1 -> If Action Subsystem/1(In1), Relational Operator/1
  If/1 -> If Action Subsystem/Action
  Constant14/1 -> Relational Operator/2
  MinMax Running Resettable1/1 -> Relational Operator1/2
  Relational Operator/1 -> Data Type Conversion/1  "t0"
  Data Type Conversion/1 -> Transport Delay/1
  In1/1 -> Relational Operator1/1, Relational Operator2/1, MinMax Running Resettable1/1
  Relational Operator2/1 -> MinMax Running Resettable1/2
  Constant/1 -> Relational Operator2/2
  If Action Subsystem/1(Out1) -> Sum/1  "picos6s"
  Sum/1 -> Product14/1
  Constant1/1 -> Sum/2

== system Monitor/Modelos de los sistemas/Respiracion/Subsystem ==
  In1 : Inport
  Clock : Clock
  Constant1 : Constant  Value=2*pi
  Constant2 : Constant  Value=1/2
  Constant3 : Constant
  Constant4 : Constant  Value=0
  Divide : Product  Inputs=*/
  Gain : Gain  Gain=1/12
  Gain1 : Gain  Gain=-1
  Product : Product
  Sin : Trigonometry
  Sum : Sum  Inputs=|+-
  Sum1 : Sum  Inputs=|++
  Switch : Switch  Criteria=u2 > Threshold
  Out1 : Outport
  wires:
  Constant1/1 -> Divide/1
  Divide/1 -> Product/2
  Constant2/1 -> Sum1/1
  Sum/1 -> Product/1
  Gain/1 -> Sum/2
  Constant3/1 -> Switch/1
  Sum1/1 -> Gain1/1
  Sin/1 -> Sum1/2
  Constant4/1 -> Switch/3
  Gain1/1 -> Switch/2
  Product/1 -> Sin/1
  In1/1 -> Divide/2, Gain/1
  Clock/1 -> Sum/1
  Switch/1 -> Out1/1

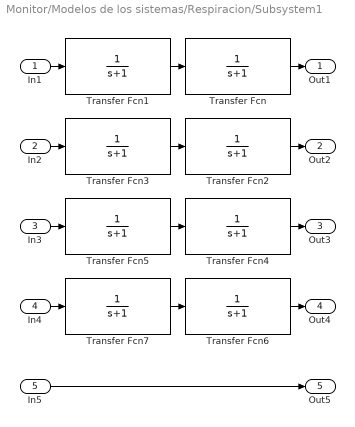
== system Monitor/Modelos de los sistemas/Respiracion/Subsystem1 ==
  In1 : Inport
  In2 : Inport  Port=2
  In3 : Inport  Port=3
  In4 : Inport  Port=4
  In5 : Inport  Port=5
  Transfer Fcn{,1..7} (8 alike) : TransferFcn  Numerator=1  Denominator=[1 1]
  Out1 : Outport
  Out2 : Outport  Port=2
  Out3 : Outport  Port=3
  Out4 : Outport  Port=4
  Out5 : Outport  Port=5
  wires:
  Transfer Fcn1/1 -> Transfer Fcn/1
  In1/1 -> Transfer Fcn1/1
  Transfer Fcn/1 -> Out1/1
  Transfer Fcn2/1 -> Out2/1
  In2/1 -> Transfer Fcn3/1
  Transfer Fcn3/1 -> Transfer Fcn2/1
  Transfer Fcn7/1 -> Transfer Fcn6/1
  In4/1 -> Transfer Fcn7/1
  Transfer Fcn6/1 -> Out4/1
  Transfer Fcn4/1 -> Out3/1
  In3/1 -> Transfer Fcn5/1
  Transfer Fcn5/1 -> Transfer Fcn4/1
  In5/1 -> Out5/1

== system Monitor/Modelos de los sistemas/Saturacion de oxigeno/Subsystem4 ==
  In1 : Inport
  Transfer Fcn : TransferFcn  Numerator=1  Denominator=[1 1]
  Transfer Fcn1 : TransferFcn  Numerator=1  Denominator=[1 1]
  Out1 : Outport
  wires:
  Transfer Fcn1/1 -> Transfer Fcn/1
  In1/1 -> Transfer Fcn1/1
  Transfer Fcn/1 -> Out1/1

== system Monitor/Modelos de los sistemas/Electrocardiograma/FrecCardiaca/If Action Subsystem ==
  In1 : Inport
  Action Port : ActionPort  ActionPortLabel=if(u1 ==1)
  Out1 : Outport
  wires:
  In1/1 -> Out1/1

== system Monitor/Modelos de los sistemas/Presion Arterial/Subsystem/Subsystem ==
  In1 : Inport
  Clock : Clock
  Constant1 : Constant  Value=2*pi
  Constant2 : Constant  Value=1/2
  Constant3 : Constant
  Constant4 : Constant  Value=0
  Divide : Product  Inputs=*/
  Gain : Gain  Gain=1/12
  Gain1 : Gain  Gain=-1
  Product : Product
  Sin : Trigonometry
  Sum : Sum  Inputs=|+-
  Sum1 : Sum  Inputs=|++
  Switch : Switch  Criteria=u2 > Threshold
  Out1 : Outport
  wires:
  Constant1/1 -> Divide/1
  Divide/1 -> Product/2
  Constant2/1 -> Sum1/1
  Sum/1 -> Product/1
  Gain/1 -> Sum/2
  Constant3/1 -> Switch/1
  Sum1/1 -> Gain1/1
  Sin/1 -> Sum1/2
  Constant4/1 -> Switch/3
  Gain1/1 -> Switch/2
  Product/1 -> Sin/1
  In1/1 -> Divide/2, Gain/1
  Clock/1 -> Sum/1
  Switch/1 -> Out1/1

== system Monitor/Modelos de los sistemas/Respiracion/Lector de frecuencia/If Action Subsystem ==
  In1 : Inport
  Action Port : ActionPort  ActionPortLabel=if(u1 ==1)
  Out1 : Outport
  wires:
  In1/1 -> Out1/1

== matlab function Monitor/datos de bebe ==
  data: datoin input; head input; nose input; caso output; abruptMov input; incubatorTemp input
function caso = fcn(datoin, head, nose, abruptMov, incubatorTemp)
    while(datoin == 0) %Saludable y mantenerlo en saludable cada que se pida
        caso = 0;
        break;
    end
    while(abruptMov==1) %siempre que se mueva abruptamente el bebe, que se agite
        caso = 3;
        break;
    end
    if(nose==2 && incubatorTemp >= 310 && abruptMov ==0 && head==0)
        caso = 1;
    end

== matlab function Monitor/caso de estudio ==
  data: crying output; u input; inTemp output; ECG output; presion output; CO2 output; ventilacion output; inOx output
function [crying, inTemp, ECG, presion, CO2, ventilacion, inOx] = fcn(u)
if u<=0 %% normal
    %TEMP
    inTemp=1;
    
    %Saturacion de oxigeno
    inOx=1;
    
    %ECG
    alphaP= 0.4; %Valor de magnitud pico onda P
    alphaQ=-5;  %Valor de magnitud pico onda Q
    picoR=18;  %Valor de magnitud pico onda R
    alphaS=-4.5; %Valor de magnitud pico onda S
    alphaT=0.25; %Valor de magnitud pico onda T
    thetaP=0.8*pi/2;
    thetaQ=pi/12;
    thetaR=0;
    thetaS=pi/12;
    thetaT = 4.5*pi/6; % Angulo donde se ubica la onda T
    omegaECG=2*pi*(138/60); %Frecuencia angular ECG
    gananciaOut= 43;  %Valor para escalar salida del modelo    
    
    %%Presion    
    Re0=0.0055222;
    Ra=0.025; 
    Rlv=0.41279; 
    Rv=0.015;
    Ce=1.69;
    Ca=2;
    Cv=7.5; 
    c1=0.01; 
    c2=4.0153; 
    c3=0.000498;
    Ed=0.0655;
    Es0=0.57; 
    epsilon=0.00001;
    A1=0.40341; 
    omega0=omegaECG;%8.37;
    offs=0;
    
    %% CO2 85-92
    phi=38; %valor max de saturacion 2:24
    %tau1=0.2; %tiempo subida inspiracion
    %tau2=0.1; %tiempo subida espiracion
    d=0.7;  %Periodo /2
    
    %% Ventilación
    Ci=9.5;
    tf = (60/36) ; %duración total del ciclo
    Vt=0.1;
    
    %% Llorar
    crying = 0;
    
elseif u==1  %%%%FIEBRE
    %Temp
    inTemp=1.075;
    
    %Saturacion de oxigeno
    inOx=0.99;
    
    %ECG
    alphaP= 0.35; %Valor de magnitud pico onda P
    alphaQ=-5;  %Valor de magnitud pico onda Q
    picoR=18;  %Valor de magnitud pico onda R
    alphaS=-3.75; %Valor de magnitud pico onda S
    alphaT=0.75*0.2; %Valor de magnitud pico onda T
    thetaP=pi/2;
    thetaQ=pi/12;
    thetaR=0;
    thetaS=pi/12;
    thetaT = 4*pi/6; % Angulo donde se ubica la onda T
    omegaECG=2*pi*(179/60); %Frecuencia angular ECG mayor a 180!!
    gananciaOut= 60; 
    
    %%Presion 85-42 aumenta para perder calor el cuero . No hipertension:
    %%esto depende de edad de peso
    Re0=0.00717;
    Ra=0.025; 
    Rlv=0.5366; 
    Rv=0.026;
    Ce=1.5210;
    Ca=1.8;
    Cv=10; 
    c1=0.01; 
    c2=4.0153;
    c3=0.000498;
    Ed=0.0655;
    Es0=0.434; 
    epsilon=0.00001; 
    A1=0.40341; 
    omega0=omegaECG;%8.37;
    offs=10;
    %% CO2 (baja saturacion)
    phi=37; %valor max de saturacion
    
    %% Ventilacion (mayor frec)
    Ci=9.5;
    tf = (60/44);%0.8; %duración total del ciclo    Tiempo inspiratorio al aumnetar frec disminuye y por eso disminuye muy poco Co2
    Vt=0.15;
    
    %Llorar
    crying = 1;
    
elseif u==2 %%%FRIO bradicardia! entre 60 y 100. Menor de 100 
    %Temp
    inTemp=0.943;
    
    %Saturacion de oxigeno
    inOx=1.01;
    
    %% ECG   
    alphaP= 0.6; %Valor de magnitud pico onda P
    alphaQ=-5;  %Valor de magnitud pico onda Q
    picoR=18;  %Valor de magnitud pico onda R
    alphaS=-7.5; %Valor de magnitud pico onda S
    alphaT=0.75*0.5; %Valor de magnitud pico onda T
    thetaP=pi/2;
    thetaQ=pi/12;
    thetaR=0;
    thetaS=pi/12;
    thetaT = 4*pi/6; % Angulo donde se ubica la onda T
    omegaECG=2*pi*(91/60); %Frecuencia angular ECG
    gananciaOut= 30;  %Valor para escalar salida del modelo 
    
    %% Presion disminuyen
    Re0=0.0055222;
    Ra=0.045; 
    Rlv=0.41279;
    Rv=0.02;
    Ce=1.859;
    Ca=2.2;
    Cv=7.5;
    c1=0.01;
    c2=4.0153;
    c3=0.000498;
    Ed=0.0655;
    Es0=0.57;
    epsilon=0.00001;
    A1=0.40341; 
    omega0=omegaECG;%8.37;
    offs=-6;
    
    %% CO2 
    phi=35; %valor max de saturacion
    
    %% Ventilacion
    Ci=0.1;
    tf = (60/29); %duración total del ciclo
    Vt=0.98;
    
    %Llorar
    crying = 1;
    
else %agitado
    %Temp
    inTemp=1;
    
    %Saturacion de oxigeno
    inOx=1;
    
    %% ECG   
    alphaP= 0.6; %Valor de magnitud pico onda P
    alphaQ=-5;  %Valor de magnitud pico onda Q
    picoR=18;  %Valor de magnitud pico onda R
    alphaS=-7.5; %Valor de magnitud pico onda S
    alphaT=0.75*0.5; %Valor de magnitud pico onda T
    thetaP=pi/2;
    thetaQ=pi/12;
    thetaR=0;
    thetaS=pi/12;
    thetaT = 4*pi/6; % Angulo donde se ubica la onda T
    omegaECG=2*pi*(145/60); %Frecuencia angular ECG
    gananciaOut= 43;  %Valor para escalar salida del modelo 
    
    %% Presion disminuyen
    Re0=0.0055222;
    Ra=0.045; 
    Rlv=0.41279;
    Rv=0.02;
    Ce=1.859;
    Ca=2.2;
    Cv=7.5;
    c1=0.01;
    c2=4.0153;
    c3=0.000498;
    Ed=0.0655;
    Es0=0.57;
    epsilon=0.00001;
    A1=0.40341; 
    omega0=omegaECG;%8.37;
    offs=0;
    
    %% Ventilación
    Ci=9.5;
    tf = (60/37); %duración total del ciclo
    Vt=0.1;
    
    %% CO2 85-92
    phi=38; %valor max de saturacion 2:24
    
    %Crying
    
    crying = 1;
  
end
Tsys= 0.3333*2*pi/omega0;
Tdia= (1-0.3333)*2*pi/omega0;
Tpresion =Tsys+Tdia;

Ri=16.41;
ti=2;  %tiempo de inspiración
A = exp(ti/(Ri*Ci));
B= exp(tf/(Ri*Ci));
Pex= -(Vt*A)/(Ci*(A-B));
D= exp(-ti/(Ri*Ci));
Pset= Pex+(Vt/(D*(A-1)*Ci));

ECG=[alphaP,alphaQ, picoR, alphaS, alphaT,thetaP, thetaQ, thetaR, thetaS, thetaT, omegaECG,gananciaOut ];
presion=[Re0, Ra, Rlv, Rv, c1, c2, c3, Ed, Ce, Ca, Cv, Es0, epsilon, A1, omega0, Tpresion, offs];
CO2=[phi,tf];
ventilacion =[Pset, Pex, tf, Ci, Vt]; %falta condicion inicial y tiempos ti tf

== stateflow chart Monitor/State Transition Table ==
  state saludable
    caso=0;
  state fiebre
    caso = 1;
  state hipotermia
    caso = 2;
  state agitado
    caso = 3
  (default) -> saludable
  saludable -> (junction 21) [order 1] : [datain == 0]
  (junction 21) -> saludable
  (junction 40) -> saludable
  (junction 42) -> (junction 40)
  saludable -> (junction 28) [order 3] : [datain == 2]
  (junction 28) -> (junction 26)
  saludable -> (junction 33) [order 4] : [datain == 3]
      | {llorar = 1;}
  (junction 33) -> (junction 73)
  saludable -> (junction 73) [order 5] : [abruptMove == 1]
      | {llorar = 1;}
  (junction 73) -> (junction 53)
  saludable -> fiebre [order 2] : [datain== 1]
  fiebre -> saludable [order 1] : [datain == 0]
  fiebre -> (junction 48) [order 2] : [datain== 1]
  (junction 48) -> fiebre
  (junction 60) -> fiebre
  (junction 62) -> (junction 60)
  fiebre -> (junction 53) [order 4] : [datain == 3]
  (junction 53) -> (junction 31)
  fiebre -> hipotermia [order 3] : [datain == 2]
  hipotermia -> fiebre [order 2] : [datain== 1]
  hipotermia -> (junction 42) [order 1] : [datain == 0]
  (junction 45) -> (junction 42)
  (junction 26) -> hipotermia
  hipotermia -> (junction 65) [order 3] : [datain == 2]
  (junction 65) -> hipotermia
  hipotermia -> agitado [order 4] : [datain == 3]
  agitado -> hipotermia [order 3] : [datain == 2]
  agitado -> (junction 45) [order 1] : [datain == 0]
  agitado -> (junction 62) [order 2] : [datain== 1]
  (junction 31) -> agitado
  agitado -> (junction 68) [order 4] : [datain == 3]
  (junction 68) -> agitado
  data: datain input; caso output; abruptMove input; llorar output
